simulink model "Outer_Loop_Linear_DCM"  (R2024b)
settings: Solver=ode15s  StartTime=0.0  StopTime=2  RelTol=1e-6  AbsTol=1e-8
undefined symbols (not defined in the file or in its folder): Ci, ctrl, DiscIntNeverNeededParam, Ts, w_start, w_stop
libraries: cstblocks x4
settings Model: SimulationMode=accelerator  Creator=rs  LastModifiedBy=overflow
settings SolverCC: AutoScaleAbsTol=off  ZeroCrossAlgorithm=Adaptive  AlgebraicLoopSolver=TrustRegion
settings DataIOCC: SaveFormat=Array  SaveOutput=off  SignalLogging=off  DSMLogging=off  SaveTime=off  ReturnWorkspaceOutputs=off  TimeSaveName=t  OutputSaveName=y
settings DebuggingCC: UnconnectedInputMsg=warning  UnconnectedOutputMsg=warning  UnconnectedLineMsg=warning  ArithmeticOperatorsInVariantConditions=warning
settings ModelReferenceCC: EnableRefExpFcnMdlSchedulingChecks=on
settings SFSimCC: SimUseLocalCustomCode=off  CustomCodeUndefinedFunction=UseInterfaceOnly
settings RTWCC: RTWUseLocalCustomCode=off  GPUComputeCapability=3.5

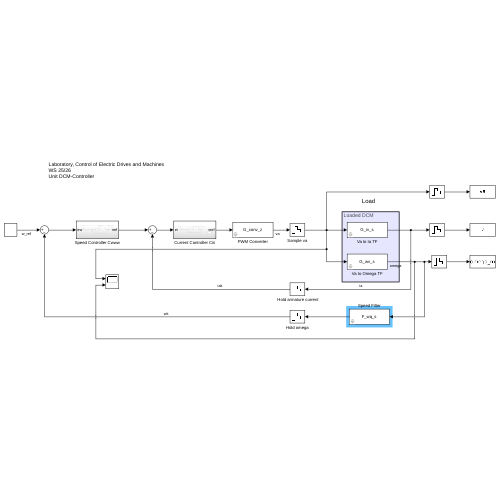
[thumbnail: Simulink's stored preview of the top-level diagram]
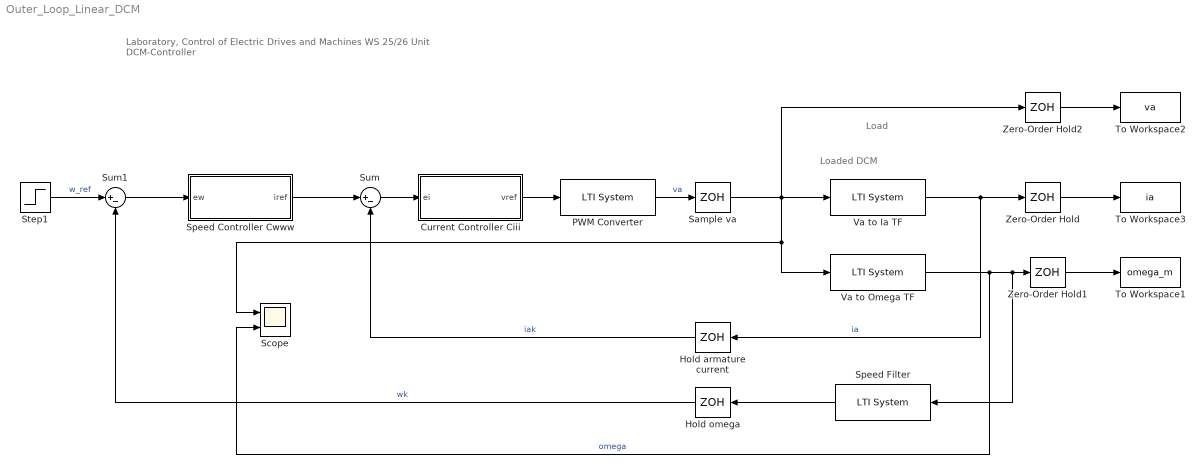
== system Outer_Loop_Linear_DCM ==
  note: Loaded DCM
  note: Laboratory, Control of Electric Drives and Machines
      | WS 25/26
      | Unit DCM-Controller
  note: Load
  " Hold armature current" : ZeroOrderHold  SampleTime=-1
  Current Controller Ciii : Subsystem
  Hold omega : ZeroOrderHold  SampleTime=-1
  PWM Converter : cstblocks/LTI System  sys=G_conv_z  IC=[]  PadeOrder=0
  Sample va : ZeroOrderHold  SampleTime=-1
  Scope : Scope  NumInputPorts=2
  Speed Controller Cwww : Subsystem
  Speed Filter : cstblocks/LTI System  sys=F_wq_s  IC=[]  PadeOrder=0
      link override Internal: InitialCondition=w_start
  Step1 : Step  Before=w_start  After=w_stop  SampleTime=0  VectorParams1D=off
  Sum : Sum  Inputs=|+-
  Sum1 : Sum  Inputs=|+-
  To Workspace1 : ToWorkspace  VariableName=omega_m  SaveFormat=Timeseries  SampleTime=-1
  To Workspace2 : ToWorkspace  VariableName=va  SaveFormat=Timeseries  SampleTime=-1
  To Workspace3 : ToWorkspace  VariableName=ia  SaveFormat=Timeseries  SampleTime=-1
  Va to Ia TF : cstblocks/LTI System  sys=G_iv_s  IC=[]  PadeOrder=0
  Va to Omega TF : cstblocks/LTI System  sys=G_wv_s  IC=[w_start 0]  PadeOrder=0
      link override Internal: InitialCondition=w_start
  Zero-Order Hold : ZeroOrderHold  SampleTime=Ts
  Zero-Order Hold1 : ZeroOrderHold  SampleTime=Ts
  Zero-Order Hold2 : ZeroOrderHold  SampleTime=Ts
  wires:
  Zero-Order Hold/1 -> To Workspace3/1
  Va to Ia TF/1 -> Zero-Order Hold/1, " Hold armature current"/1  "ia"
  Zero-Order Hold2/1 -> To Workspace2/1
  Sum/1 -> Current Controller Ciii/1(ei)
  " Hold armature current"/1 -> Sum/2  "iak"
  Speed Controller Cwww/1(iref) -> Sum/1
  Sample va/1 -> Va to Omega TF/1, Scope/1, Va to Ia TF/1, Zero-Order Hold2/1
  PWM Converter/1 -> Sample va/1  "va"
  Current Controller Ciii/1(vref) -> PWM Converter/1
  Zero-Order Hold1/1 -> To Workspace1/1
  Va to Omega TF/1 -> Scope/2, Speed Filter/1, Zero-Order Hold1/1  "omega"
  Sum1/1 -> Speed Controller Cwww/1(ew)
  Step1/1 -> Sum1/1  "w_ref"
  Hold omega/1 -> Sum1/2  "wk"
  Speed Filter/1 -> Hold omega/1

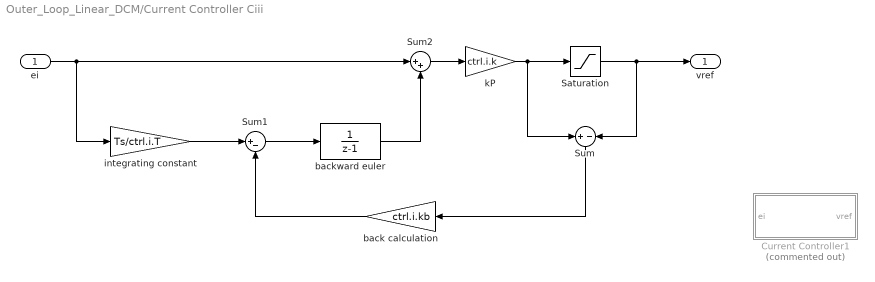
== system Outer_Loop_Linear_DCM/Current Controller Ciii ==
  ei : Inport
  Current Controller1 : Subsystem  Commented=on
  Saturation : Saturate  UpperLimit=ctrl.i.satP  LowerLimit=ctrl.i.satN
  Sum : Sum  Inputs=+|-
  Sum1 : Sum  Inputs=|+-
  Sum2 : Sum  Inputs=|++
  back calculation : Gain  Gain=ctrl.i.kb
  backward euler : DiscreteTransferFcn  Denominator=[1 -1]
  integrating constant : Gain  Gain=Ts/ctrl.i.T
  kP : Gain  Gain=ctrl.i.k
  vref : Outport
  wires:
  Sum1/1 -> backward euler/1
  integrating constant/1 -> Sum1/1
  Saturation/1 -> vref/1, Sum/2
  Sum/1 -> back calculation/1
  back calculation/1 -> Sum1/2
  ei/1 -> integrating constant/1, Sum2/1
  Sum2/1 -> kP/1
  kP/1 -> Sum/1, Saturation/1
  backward euler/1 -> Sum2/2

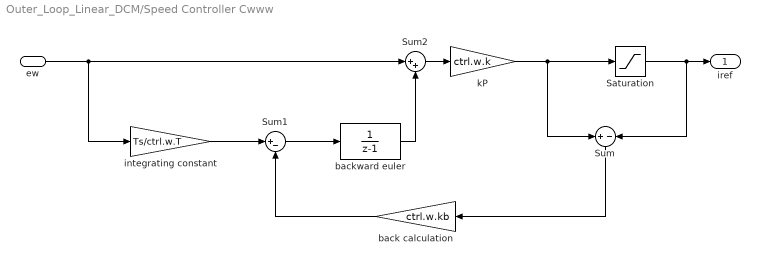
== system Outer_Loop_Linear_DCM/Speed Controller Cwww ==
  ew : Inport
  Saturation : Saturate  UpperLimit=ctrl.w.satP  LowerLimit=ctrl.w.satN
  Sum : Sum  Inputs=+|-
  Sum1 : Sum  Inputs=|+-
  Sum2 : Sum  Inputs=|++
  back calculation : Gain  Gain=ctrl.w.kb
  backward euler : DiscreteTransferFcn  Denominator=[1 -1]
  integrating constant : Gain  Gain=Ts/ctrl.w.T
  kP : Gain  Gain=ctrl.w.k
  iref : Outport
  wires:
  ew/1 -> Sum2/1, integrating constant/1
  backward euler/1 -> Sum2/2
  Saturation/1 -> iref/1, Sum/2
  back calculation/1 -> Sum1/2
  integrating constant/1 -> Sum1/1
  Sum/1 -> back calculation/1
  kP/1 -> Sum/1, Saturation/1
  Sum2/1 -> kP/1
  Sum1/1 -> backward euler/1

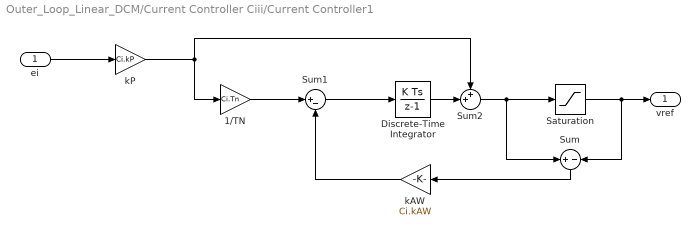
== system Outer_Loop_Linear_DCM/Current Controller Ciii/Current Controller1 ==
  ei : Inport
  1/TN : Gain  Gain=Ci.Tn
  Discrete-Time Integrator : DiscreteIntegrator  SampleTime=-1  ICPrevOutput=DiscIntNeverNeededParam  ICPrevScaledInput=DiscIntNeverNeededParam
  Saturation : Saturate
  Sum : Sum  Inputs=+|-
  Sum1 : Sum  Inputs=|+-
  Sum2 : Sum  Inputs=++|
  kAW : Gain  Gain=Ci.kAW
  kP : Gain  Gain=Ci.kP
  vref : Outport
  wires:
  Sum1/1 -> Discrete-Time Integrator/1
  1/TN/1 -> Sum1/1
  Discrete-Time Integrator/1 -> Sum2/2
  ei/1 -> kP/1
  Sum2/1 -> Sum/1, Saturation/1
  Saturation/1 -> Sum/2, vref/1
  Sum/1 -> kAW/1
  kAW/1 -> Sum1/2
  kP/1 -> Sum2/1, 1/TN/1
